simulink model "Jenkins_Brake"  (R2021a)
settings: Solver=ode1  StartTime=0.0  StopTime=inf  FixedStep=0.001  RelTol=1e-3
PreLoadFcn:
  | vehicle = 'Car'; if ~length(which('cmself')), cmenv; end
  | Jenkins_Brake_bus
InitFcn:
  | vehicle = 'Car'; if ~length(which('cmself')), cmenv; end
  | Jenkins_Brake_bus
Description:
  | CarMaker Plug-in Model Target
settings Model: Creator=giri  LastModifiedBy=giri
settings RTWCC: Description=CarMaker Plug-in Model Target  SystemTargetFile=CarMaker.tlc  TemplateMakefile=CarMaker_unix-linux64.tmf
settings CodeAppCC: MaxIdLength=127
settings STFCustomTargetCC: TargetLangStandard=C99 (ISO)  CombineOutputUpdateFcns=on  CodeInterfacePackaging=Reusable function  GRTInterface=off  GenerateAllocFcn=on  UseToolchainInfoCompliant=off  SystemTargetFile=CarMaker.tlc
settings GRTTargetCC: ParMdlRefBuildCompliant=off  CompOptLevelCompliant=off  ConcurrentExecutionCompliant=off  MatFileLogging=off  CodeInterfacePackaging=Reusable function  CPPClassGenCompliant=off  GenerateAllocFcn=on  UseToolchainInfoCompliant=off

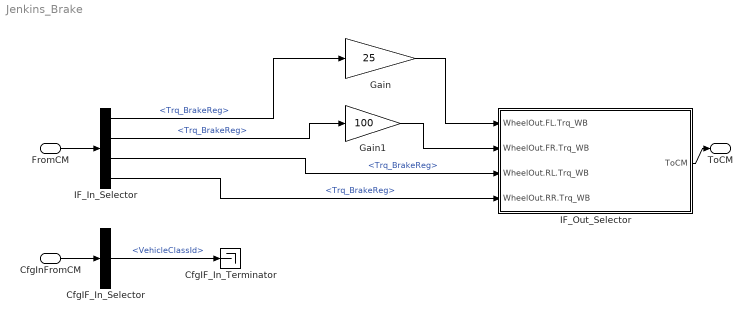
== system Jenkins_Brake ==
  FromCM : Inport  OutDataTypeStr=Bus: cmBrakeIn
  CfgInFromCM : Inport  Port=2  OutDataTypeStr=Bus: cmBrakeCfgIn
  CfgIF_In_Selector : BusSelector  OutputSignals=VehicleClassId
  CfgIF_In_Terminator : Terminator
  Gain : Gain  Gain=25
  Gain1 : Gain  Gain=100
  IF_In_Selector : BusSelector  OutputSignals=WheelIn.RR.Trq_BrakeReg,WheelIn.RL.Trq_BrakeReg,WheelIn.FR.Trq_BrakeReg,WheelIn.FL.Trq_BrakeReg
  IF_Out_Selector : Subsystem  mask(Signal Selection){}
      mask help: Signal Selection Block
      settings: OpenFcn=cmSignalSelect('SignalSelection_CB',gcb)
  ToCM : Outport  OutDataTypeStr=Bus: cmBrakeOut
  wires:
  FromCM/1 -> IF_In_Selector/1
  IF_In_Selector/1 -> Gain/1  "<Trq_BrakeReg>"
  IF_Out_Selector/1(ToCM) -> ToCM/1
  CfgInFromCM/1 -> CfgIF_In_Selector/1
  CfgIF_In_Selector/1 -> CfgIF_In_Terminator/1  "<VehicleClassId>"
  IF_In_Selector/2 -> Gain1/1  "<Trq_BrakeReg>"
  IF_In_Selector/3 -> IF_Out_Selector/3(WheelOut.RL.Trq_WB)  "<Trq_BrakeReg>"
  IF_In_Selector/4 -> IF_Out_Selector/4(WheelOut.RR.Trq_WB)  "<Trq_BrakeReg>"
  Gain/1 -> IF_Out_Selector/1(WheelOut.FL.Trq_WB)
  Gain1/1 -> IF_Out_Selector/2(WheelOut.FR.Trq_WB)

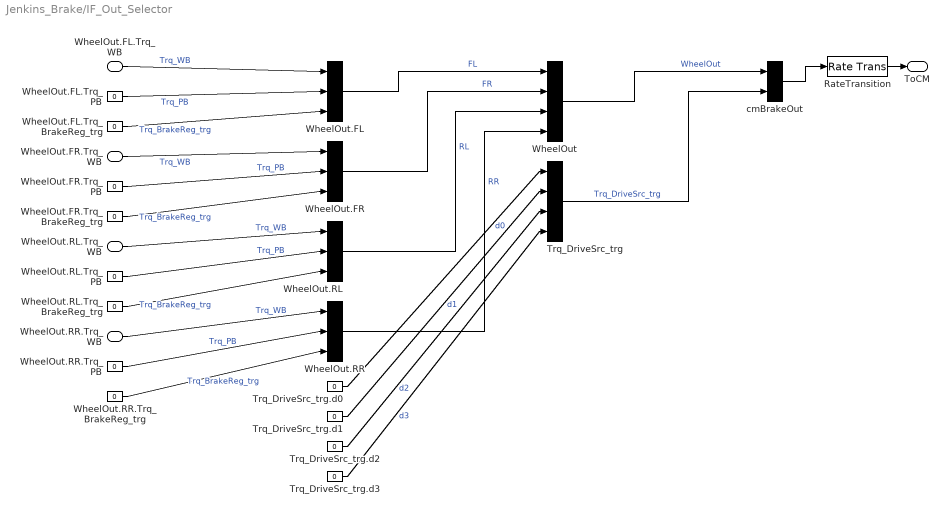
== system Jenkins_Brake/IF_Out_Selector ==
  WheelOut.FL.Trq_WB : Inport
  WheelOut.FR.Trq_WB : Inport  Port=2
  WheelOut.RL.Trq_WB : Inport  Port=3
  WheelOut.RR.Trq_WB : Inport  Port=4
  RateTransition : RateTransition  OutPortSampleTime=str2num(get_param(bdroot,'FixedStep'))
  Trq_DriveSrc_trg : BusCreator  Inputs=4
  Trq_DriveSrc_trg.d{0..3} (4 alike) : Constant  Value=0
  WheelOut : BusCreator  Inputs=4
  WheelOut.FL : BusCreator  Inputs=3
  WheelOut.FL.Trq_BrakeReg_trg : Constant  Value=0
  WheelOut.FL.Trq_PB : Constant  Value=0
  WheelOut.FR : BusCreator  Inputs=3
  WheelOut.FR.Trq_BrakeReg_trg : Constant  Value=0
  WheelOut.FR.Trq_PB : Constant  Value=0
  WheelOut.RL : BusCreator  Inputs=3
  WheelOut.RL.Trq_BrakeReg_trg : Constant  Value=0
  WheelOut.RL.Trq_PB : Constant  Value=0
  WheelOut.RR : BusCreator  Inputs=3
  WheelOut.RR.Trq_BrakeReg_trg : Constant  Value=0
  WheelOut.RR.Trq_PB : Constant  Value=0
  cmBrakeOut : BusCreator  Inputs=2
  ToCM : Outport
  wires:
  RateTransition/1 -> ToCM/1
  cmBrakeOut/1 -> RateTransition/1
  WheelOut/1 -> cmBrakeOut/1  "WheelOut"
  WheelOut.FL/1 -> WheelOut/1  "FL"
  WheelOut.FL.Trq_PB/1 -> WheelOut.FL/2  "Trq_PB"
  WheelOut.FL.Trq_BrakeReg_trg/1 -> WheelOut.FL/3  "Trq_BrakeReg_trg"
  WheelOut.FR/1 -> WheelOut/2  "FR"
  WheelOut.FR.Trq_PB/1 -> WheelOut.FR/2  "Trq_PB"
  WheelOut.FR.Trq_BrakeReg_trg/1 -> WheelOut.FR/3  "Trq_BrakeReg_trg"
  WheelOut.RL/1 -> WheelOut/3  "RL"
  WheelOut.RL.Trq_PB/1 -> WheelOut.RL/2  "Trq_PB"
  WheelOut.RL.Trq_BrakeReg_trg/1 -> WheelOut.RL/3  "Trq_BrakeReg_trg"
  WheelOut.RR/1 -> WheelOut/4  "RR"
  WheelOut.RR.Trq_PB/1 -> WheelOut.RR/2  "Trq_PB"
  WheelOut.RR.Trq_BrakeReg_trg/1 -> WheelOut.RR/3  "Trq_BrakeReg_trg"
  Trq_DriveSrc_trg/1 -> cmBrakeOut/2  "Trq_DriveSrc_trg"
  Trq_DriveSrc_trg.d0/1 -> Trq_DriveSrc_trg/1  "d0"
  Trq_DriveSrc_trg.d1/1 -> Trq_DriveSrc_trg/2  "d1"
  Trq_DriveSrc_trg.d2/1 -> Trq_DriveSrc_trg/3  "d2"
  Trq_DriveSrc_trg.d3/1 -> Trq_DriveSrc_trg/4  "d3"
  WheelOut.FL.Trq_WB/1 -> WheelOut.FL/1  "Trq_WB"
  WheelOut.FR.Trq_WB/1 -> WheelOut.FR/1  "Trq_WB"
  WheelOut.RL.Trq_WB/1 -> WheelOut.RL/1  "Trq_WB"
  WheelOut.RR.Trq_WB/1 -> WheelOut.RR/1  "Trq_WB"
